simulink model "p3"  (R2015a)
settings: Solver=ode4  StartTime=0.0  StopTime=30  FixedStep=0.01  RelTol=1e-3
values from neighbouring files (symbols this model uses):
  g = 9.81    [env.m]
  K = [2*g; 1]    [env.m]
  l = 10    [env.m]
  ue = 0    [env.m]
  x0 = [pi/2 0]    [env.m]
  xe = [0; 0]    [env.m]
libraries: simulink x1
settings Model: Creator=jgutierr  LastModifiedBy=vdrouinv

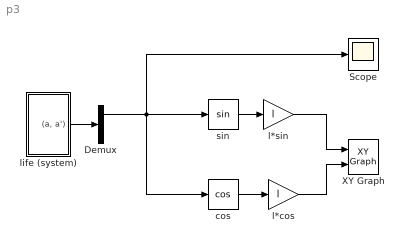
== system p3 ==
  Demux : Demux  Outputs=2
  Scope : Scope
  XY Graph : simulink/Sinks/XY Graph  xmin=-10  xmax=10  ymin=-10  ymax=10  st=-1
  cos : Trigonometry  Operator=cos
  l*cos : Gain  Gain=l
  l*sin : Gain  Gain=l
  life (system) : Subsystem
  sin : Trigonometry
  wires:
  l*sin/1 -> XY Graph/1
  l*cos/1 -> XY Graph/2
  cos/1 -> l*cos/1
  sin/1 -> l*sin/1
  Demux/1 -> Scope/1, sin/1, cos/1
  life (system)/1("(a, a')") -> Demux/1

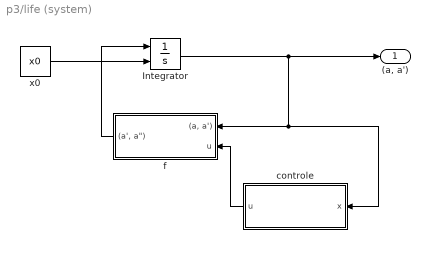
== system p3/life (system) ==
  Integrator : Integrator  InitialConditionSource=external
  controle : Subsystem  TreatAsAtomicUnit=on
  f : Subsystem
  x0 : Constant  Value=x0
  "(a, a')" : Outport
  wires:
  x0/1 -> Integrator/2
  f/1("(a', a\")") -> Integrator/1
  Integrator/1 -> "(a, a')"/1, controle/1(x), f/1("(a, a')")
  controle/1(u) -> f/2(u)

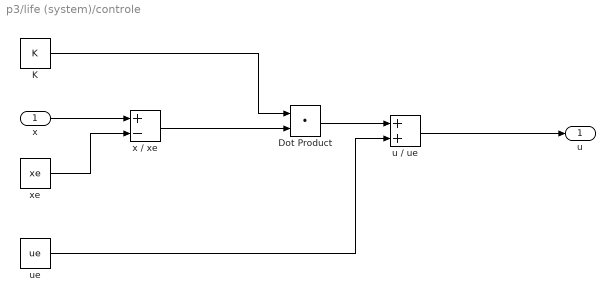
== system p3/life (system)/controle ==
  x : Inport
  Dot Product : DotProduct  InputSameDT=on  OutDataTypeStr=Inherit: Inherit via internal rule
  K : Constant  Value=K
  u / ue : Sum
  ue : Constant  Value=ue
  x / xe : Sum  Inputs=+-
  xe : Constant  Value=xe
  u : Outport
  wires:
  x/1 -> x / xe/1
  xe/1 -> x / xe/2
  x / xe/1 -> Dot Product/2
  K/1 -> Dot Product/1
  Dot Product/1 -> u / ue/1
  ue/1 -> u / ue/2
  u / ue/1 -> u/1

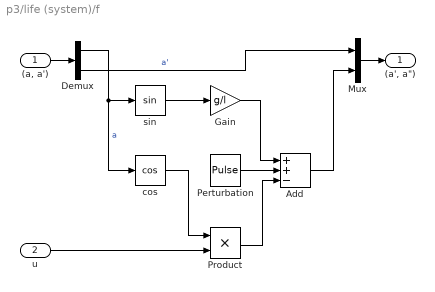
== system p3/life (system)/f ==
  "(a, a')" : Inport
  u : Inport  Port=2
  Add : Sum  Inputs=++-
  Demux : Demux  Outputs=2
  Gain : Gain  Gain=g/l
  Mux : Mux  Inputs=2
  Perturbation : DiscretePulseGenerator  PulseType=Time based  Amplitude=10  Period=10
  Product : Product
  cos : Trigonometry  Operator=cos
  sin : Trigonometry
  "(a', a\")" : Outport
  wires:
  Gain/1 -> Add/1
  Demux/1 -> cos/1, sin/1  "a"
  Demux/2 -> Mux/1  "a'"
  sin/1 -> Gain/1
  "(a, a')"/1 -> Demux/1
  Mux/1 -> "(a', a\")"/1
  cos/1 -> Product/1
  u/1 -> Product/2
  Perturbation/1 -> Add/2
  Product/1 -> Add/3
  Add/1 -> Mux/2
